simulink model "LQR"  (R2023a)
settings: Solver=VariableStepAuto  StartTime=0.0  StopTime=1  RelTol=1e-3
values from neighbouring files (symbols this model uses):
  A_val = cell(1,3)    [codex.m]
  B_val = cell(1,3)    [codex.m]
  C = [0 1]    [codex.m]
  K_val = cell(1,3)    [codex.m]
settings Model: Creator=Hi  LastModifiedBy=Hi

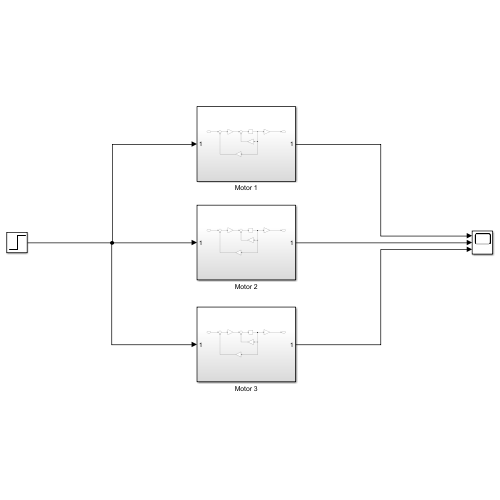
[thumbnail: Simulink's stored preview of the top-level diagram]
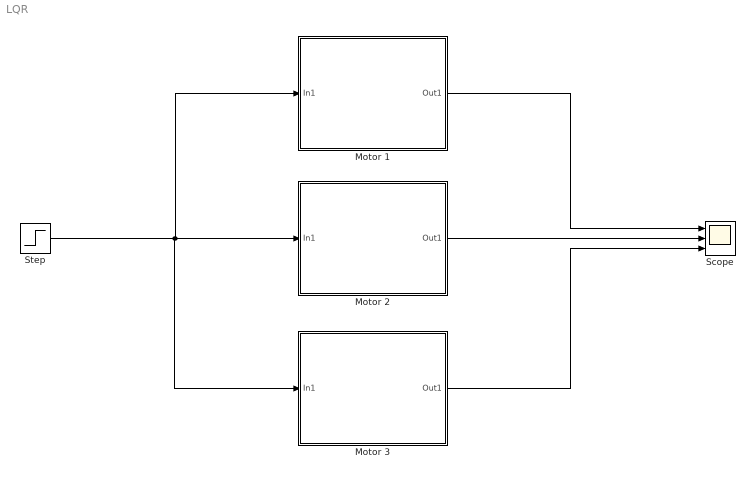
== system LQR ==
  Motor 1 : Subsystem
  Motor 2 : Subsystem
  Motor 3 : Subsystem
  Scope : Scope  NumInputPorts=3
  Step : Step  Time=0.1  SampleTime=0
  wires:
  Step/1 -> Motor 3/1(In1), Motor 2/1(In1), Motor 1/1(In1)
  Motor 1/1(Out1) -> Scope/1
  Motor 2/1(Out1) -> Scope/2
  Motor 3/1(Out1) -> Scope/3

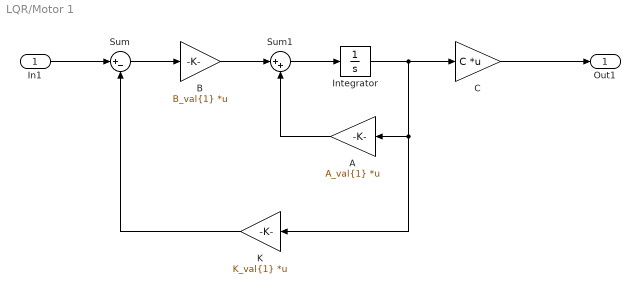
== system LQR/Motor 1 ==
  In1 : Inport
  A : Gain  Gain=A_val{1}  Multiplication=Matrix(K*u)
  B : Gain  Gain=B_val{1}  Multiplication=Matrix(K*u)
  C : Gain  Gain=C  Multiplication=Matrix(K*u)
  Integrator : Integrator
  K : Gain  Gain=K_val{1}  Multiplication=Matrix(K*u)
  Sum : Sum  Inputs=|+-
  Sum1 : Sum  Inputs=|++
  Out1 : Outport
  wires:
  Integrator/1 -> K/1, A/1, C/1
  Sum/1 -> B/1
  K/1 -> Sum/2
  A/1 -> Sum1/2
  B/1 -> Sum1/1
  In1/1 -> Sum/1
  Sum1/1 -> Integrator/1
  C/1 -> Out1/1

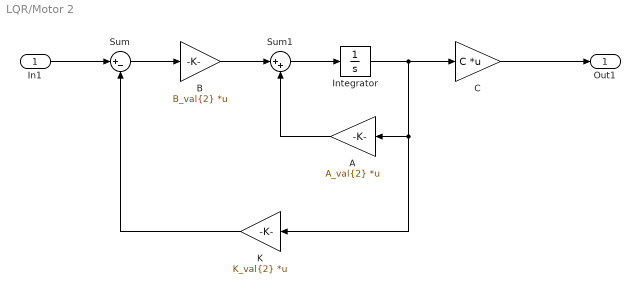
== system LQR/Motor 2 ==
  In1 : Inport
  A : Gain  Gain=A_val{2}  Multiplication=Matrix(K*u)
  B : Gain  Gain=B_val{2}  Multiplication=Matrix(K*u)
  C : Gain  Gain=C  Multiplication=Matrix(K*u)
  Integrator : Integrator
  K : Gain  Gain=K_val{2}  Multiplication=Matrix(K*u)
  Sum : Sum  Inputs=|+-
  Sum1 : Sum  Inputs=|++
  Out1 : Outport
  wires:
  Integrator/1 -> K/1, A/1, C/1
  Sum/1 -> B/1
  K/1 -> Sum/2
  A/1 -> Sum1/2
  B/1 -> Sum1/1
  In1/1 -> Sum/1
  Sum1/1 -> Integrator/1
  C/1 -> Out1/1

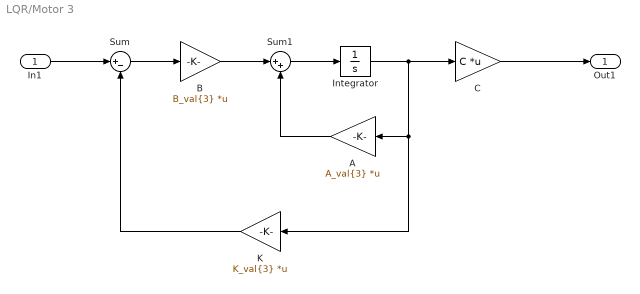
== system LQR/Motor 3 ==
  In1 : Inport
  A : Gain  Gain=A_val{3}  Multiplication=Matrix(K*u)
  B : Gain  Gain=B_val{3}  Multiplication=Matrix(K*u)
  C : Gain  Gain=C  Multiplication=Matrix(K*u)
  Integrator : Integrator
  K : Gain  Gain=K_val{3}  Multiplication=Matrix(K*u)
  Sum : Sum  Inputs=|+-
  Sum1 : Sum  Inputs=|++
  Out1 : Outport
  wires:
  Integrator/1 -> K/1, A/1, C/1
  Sum/1 -> B/1
  K/1 -> Sum/2
  A/1 -> Sum1/2
  B/1 -> Sum1/1
  In1/1 -> Sum/1
  Sum1/1 -> Integrator/1
  C/1 -> Out1/1
